simulink model "ESTS_FRIC_SLIP_test"  (R2024b)
settings: Solver=VariableStepAuto  StartTime=0.0  StopTime=10.0  RelTol=1e-3
libraries: ESTS_FRIC_SLIP x1
settings Model: Creator=blatak  LastModifiedBy=blatak

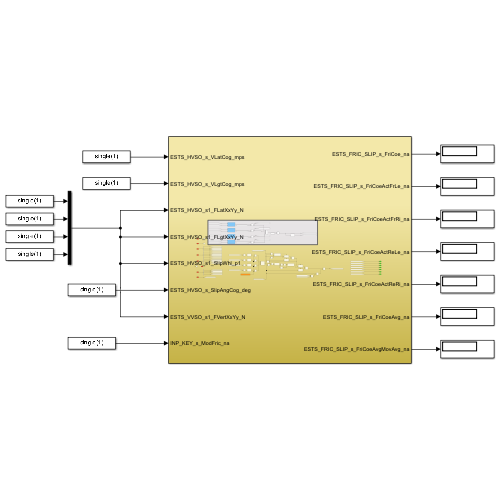
[thumbnail: Simulink's stored preview of the top-level diagram]
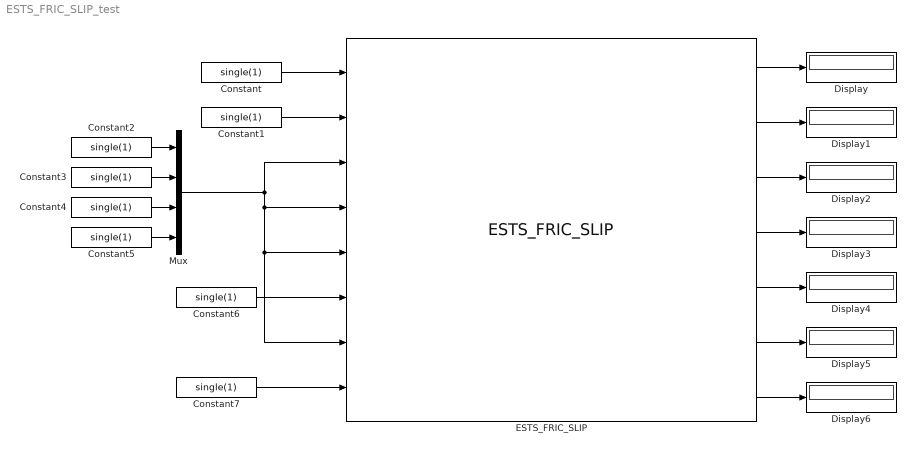
== system ESTS_FRIC_SLIP_test ==
  Constant{,1..7} (8 alike) : Constant  Value=single(1)
  Display{,1..6} (7 alike) : Display
  ESTS_FRIC_SLIP : ESTS_FRIC_SLIP/ESTS_FRIC_SLIP  SystemSampleTime=-1  VariantActivationTime=update diagram  AllowFlexibleInterface=on  Latency=0  AutoFrameSizeCalculation=off
  Mux : Mux
  wires:
  Constant/1 -> ESTS_FRIC_SLIP/1
  Constant1/1 -> ESTS_FRIC_SLIP/2
  Constant2/1 -> Mux/1
  Constant3/1 -> Mux/2
  Constant4/1 -> Mux/3
  Constant5/1 -> Mux/4
  Mux/1 -> ESTS_FRIC_SLIP/3, ESTS_FRIC_SLIP/7, ESTS_FRIC_SLIP/5, ESTS_FRIC_SLIP/4
  Constant6/1 -> ESTS_FRIC_SLIP/6
  Constant7/1 -> ESTS_FRIC_SLIP/8
  ESTS_FRIC_SLIP/1 -> Display/1
  ESTS_FRIC_SLIP/2 -> Display1/1
  ESTS_FRIC_SLIP/3 -> Display2/1
  ESTS_FRIC_SLIP/4 -> Display3/1
  ESTS_FRIC_SLIP/5 -> Display4/1
  ESTS_FRIC_SLIP/6 -> Display5/1
  ESTS_FRIC_SLIP/7 -> Display6/1
